simulink model "Battery_Dataset_Generator"  (R2024b)
settings: Solver=FixedStepDiscrete  StartTime=0.0  StopTime=25000  FixedStep=1  RelTol=1e-3
libraries: simulink x1
settings Model: Creator=karth  LastModifiedBy=karth

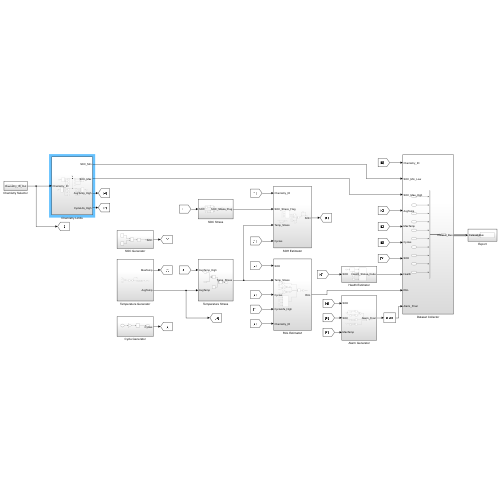
[thumbnail: Simulink's stored preview of the top-level diagram]
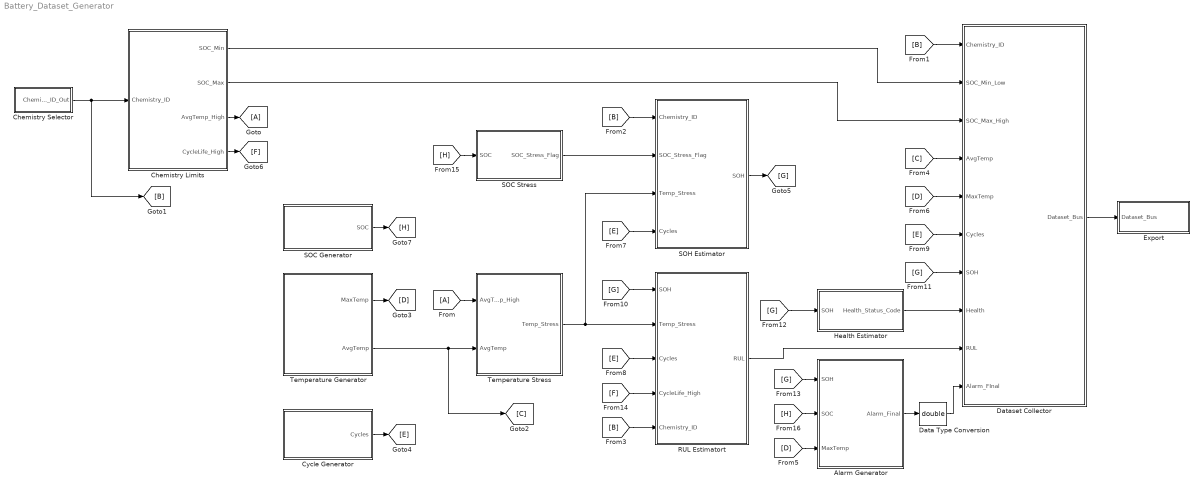
== system Battery_Dataset_Generator ==
  Alarm Generator : Subsystem
  Chemistry Limits : Subsystem
  Chemistry Selector : Subsystem
  Cycle Generator : Subsystem
  Data Type Conversion : DataTypeConversion  OutDataTypeStr=double  SaturateOnIntegerOverflow=off  RndMeth=Floor
  Dataset Collector : Subsystem
  Export : Subsystem
  From : From
  Goto : Goto
  Health Estimator : Subsystem
  RUL Estimatort : Subsystem
  SOC Generator : Subsystem
  SOC Stress : Subsystem
  SOH Estimator : Subsystem
  Temperature Generator : Subsystem
  Temperature Stress : Subsystem
  wires:
  Dataset Collector/1(Dataset_Bus) -> Export/1(Dataset_Bus)
  Chemistry Selector/1(Chemistry_ID_Out) -> Chemistry Limits/1(Chemistry_ID), [B]
  SOC Stress/1(SOC_Stress_Flag) -> SOH Estimator/2(SOC_Stress_Flag)
  Temperature Stress/1(Temp_Stress) -> SOH Estimator/3(Temp_Stress), RUL Estimatort/2(Temp_Stress)
  Chemistry Limits/1(SOC_Min) -> Dataset Collector/2(SOC_Min_Low)
  Chemistry Limits/2(SOC_Max) -> Dataset Collector/3(SOC_Max_High)
  Temperature Generator/2(AvgTemp) -> [C], Temperature Stress/2(AvgTemp)
  RUL Estimatort/1(RUL) -> Dataset Collector/9(RUL)
  Health Estimator/1(Health_Status_Code) -> Dataset Collector/8(Health)
  Chemistry Limits/3(AvgTemp_High) -> Goto/1
  From/1 -> Temperature Stress/1(AvgTemp_High)
  [B] -> SOH Estimator/1(Chemistry_ID)
  [B] -> Dataset Collector/1(Chemistry_ID)
  [C] -> Dataset Collector/4(AvgTemp)
  Temperature Generator/1(MaxTemp) -> [D]
  [D] -> Alarm Generator/3(MaxTemp)
  [D] -> Dataset Collector/5(MaxTemp)
  Cycle Generator/1(Cycles) -> [E]
  [E] -> SOH Estimator/4(Cycles)
  [E] -> RUL Estimatort/3(Cycles)
  [E] -> Dataset Collector/6(Cycles)
  [B] -> RUL Estimatort/5(Chemistry_ID)
  SOH Estimator/1(SOH) -> [G]
  [G] -> Dataset Collector/7(SOH)
  [G] -> Alarm Generator/1(SOH)
  [G] -> Health Estimator/1(SOH)
  [G] -> RUL Estimatort/1(SOH)
  Chemistry Limits/4(CycleLife_High) -> [F]
  [F] -> RUL Estimatort/4(CycleLife_High)
  SOC Generator/1(SOC) -> [H]
  [H] -> SOC Stress/1(SOC)
  [H] -> Alarm Generator/2(SOC)
  Alarm Generator/1(Alarm_Final) -> Data Type Conversion/1
  Data Type Conversion/1 -> Dataset Collector/10(Alarm_FInal)

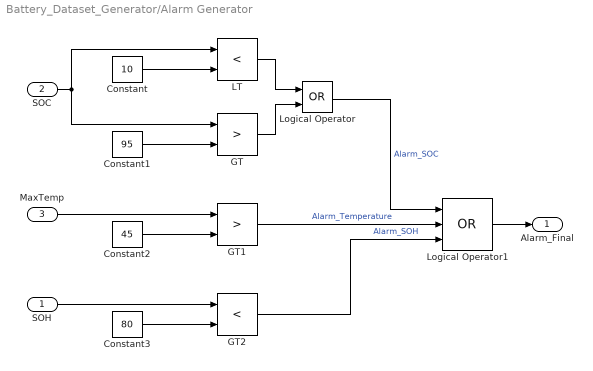
== system Battery_Dataset_Generator/Alarm Generator ==
  SOH : Inport
  SOC : Inport  Port=2
  MaxTemp : Inport  Port=3
  Constant : Constant  Value=10
  Constant1 : Constant  Value=95
  Constant2 : Constant  Value=45
  Constant3 : Constant  Value=80
  GT : RelationalOperator  Operator=>  OutDataTypeStr=boolean  RndMeth=Simplest  InputSameDT=off
  GT1 : RelationalOperator  Operator=>  OutDataTypeStr=boolean  RndMeth=Simplest  InputSameDT=off
  GT2 : RelationalOperator  Operator=<  OutDataTypeStr=boolean  RndMeth=Simplest  InputSameDT=off
  LT : RelationalOperator  Operator=<  OutDataTypeStr=boolean  RndMeth=Simplest  InputSameDT=off
  Logical Operator : Logic  Operator=OR  AllPortsSameDT=off  OutDataTypeStr=boolean
  Logical Operator1 : Logic  Operator=OR  Inputs=3  AllPortsSameDT=off  OutDataTypeStr=boolean
  Alarm_Final : Outport
  wires:
  Constant1/1 -> GT/2
  LT/1 -> Logical Operator/1
  GT/1 -> Logical Operator/2
  SOC/1 -> GT/1, LT/1
  Logical Operator/1 -> Logical Operator1/1  "Alarm_SOC"
  Constant/1 -> LT/2
  GT1/1 -> Logical Operator1/2  "Alarm_Temperature"
  Constant2/1 -> GT1/2
  MaxTemp/1 -> GT1/1
  Constant3/1 -> GT2/2
  GT2/1 -> Logical Operator1/3  "Alarm_SOH"
  SOH/1 -> GT2/1
  Logical Operator1/1 -> Alarm_Final/1

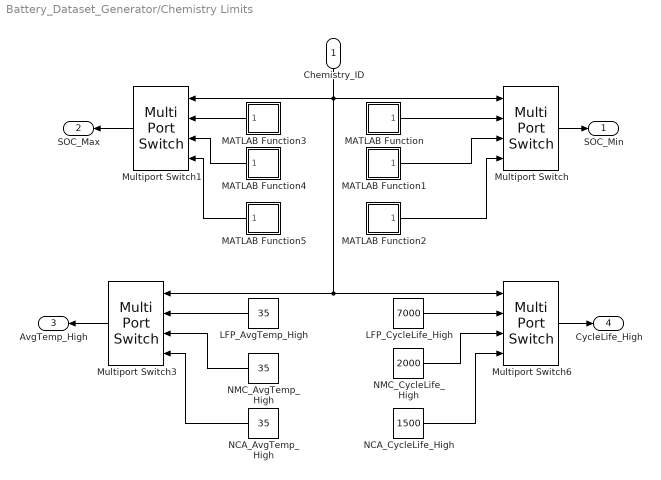
== system Battery_Dataset_Generator/Chemistry Limits ==
  Chemistry_ID : Inport
  LFP_AvgTemp_High : Constant  Value=35
  LFP_CycleLife_High : Constant  Value=7000
  MATLAB Function : MATLAB Function  TreatAsAtomicUnit=on
  MATLAB Function1 : MATLAB Function  TreatAsAtomicUnit=on
  MATLAB Function2 : MATLAB Function  TreatAsAtomicUnit=on
  MATLAB Function3 : MATLAB Function  TreatAsAtomicUnit=on
  MATLAB Function4 : MATLAB Function  TreatAsAtomicUnit=on
  MATLAB Function5 : MATLAB Function  TreatAsAtomicUnit=on
  Multiport Switch{,1,3,6} (4 alike) : MultiPortSwitch  SaturateOnIntegerOverflow=off  InputSameDT=off
  NCA_AvgTemp_High : Constant  Value=35
  NCA_CycleLife_High : Constant  Value=1500
  NMC_AvgTemp_High : Constant  Value=35
  NMC_CycleLife_High : Constant  Value=2000
  SOC_Min : Outport
  SOC_Max : Outport  Port=2
  AvgTemp_High : Outport  Port=3
  CycleLife_High : Outport  Port=4
  wires:
  Multiport Switch/1 -> SOC_Min/1
  Multiport Switch1/1 -> SOC_Max/1
  Multiport Switch3/1 -> AvgTemp_High/1
  MATLAB Function/1(soc_max) -> Multiport Switch/2
  MATLAB Function1/1(soc_max) -> Multiport Switch/3
  MATLAB Function2/1(soc_max) -> Multiport Switch/4
  Chemistry_ID/1 -> Multiport Switch6/1, Multiport Switch3/1, Multiport Switch1/1, Multiport Switch/1
  NCA_AvgTemp_High/1 -> Multiport Switch3/4
  NMC_AvgTemp_High/1 -> Multiport Switch3/3
  LFP_AvgTemp_High/1 -> Multiport Switch3/2
  NMC_CycleLife_High/1 -> Multiport Switch6/3
  Multiport Switch6/1 -> CycleLife_High/1
  LFP_CycleLife_High/1 -> Multiport Switch6/2
  NCA_CycleLife_High/1 -> Multiport Switch6/4
  MATLAB Function3/1(soc_min) -> Multiport Switch1/2
  MATLAB Function4/1(soc_min) -> Multiport Switch1/3
  MATLAB Function5/1(soc_min) -> Multiport Switch1/4

== system Battery_Dataset_Generator/Chemistry Selector ==
  Chemistry_Profile : FromWorkspace  VariableName=chem_profile  SampleTime=1
  Chemistry_ID_Out : Outport
  wires:
  Chemistry_Profile/1 -> Chemistry_ID_Out/1

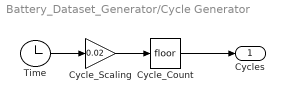
== system Battery_Dataset_Generator/Cycle Generator ==
  Cycle_Count : Rounding
  Cycle_Scaling : Gain  Gain=0.02
  Time : Clock
  Cycles : Outport
  wires:
  Time/1 -> Cycle_Scaling/1
  Cycle_Scaling/1 -> Cycle_Count/1
  Cycle_Count/1 -> Cycles/1

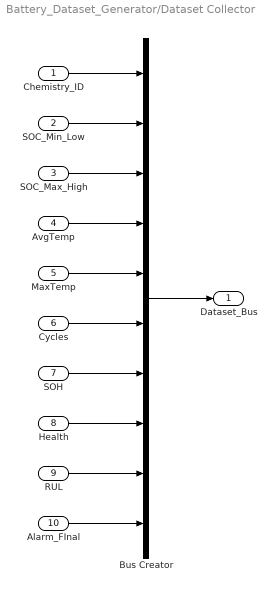
== system Battery_Dataset_Generator/Dataset Collector ==
  Chemistry_ID : Inport
  SOC_Min_Low : Inport  Port=2
  SOC_Max_High : Inport  Port=3
  AvgTemp : Inport  Port=4
  MaxTemp : Inport  Port=5
  Cycles : Inport  Port=6
  SOH : Inport  Port=7
  Health : Inport  Port=8
  RUL : Inport  Port=9
  Alarm_FInal : Inport  Port=10
  Bus Creator : BusCreator  Inputs=10
  Dataset_Bus : Outport
  wires:
  Chemistry_ID/1 -> Bus Creator/1
  SOC_Min_Low/1 -> Bus Creator/2
  SOC_Max_High/1 -> Bus Creator/3
  AvgTemp/1 -> Bus Creator/4
  MaxTemp/1 -> Bus Creator/5
  Cycles/1 -> Bus Creator/6
  SOH/1 -> Bus Creator/7
  Health/1 -> Bus Creator/8
  RUL/1 -> Bus Creator/9
  Alarm_FInal/1 -> Bus Creator/10
  Bus Creator/1 -> Dataset_Bus/1

== system Battery_Dataset_Generator/Export ==
  Dataset_Bus : Inport
  To Workspace : ToWorkspace  VariableName=evbattery  SaveFormat=Structure With Time  SampleTime=1
  wires:
  Dataset_Bus/1 -> To Workspace/1

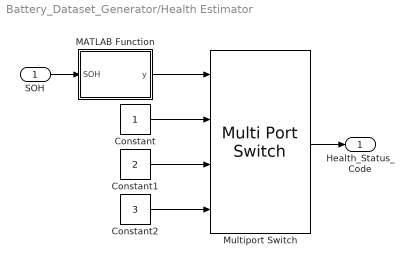
== system Battery_Dataset_Generator/Health Estimator ==
  SOH : Inport
  Constant : Constant
  Constant1 : Constant  Value=2
  Constant2 : Constant  Value=3
  MATLAB Function : MATLAB Function  TreatAsAtomicUnit=on
  Multiport Switch : MultiPortSwitch  SaturateOnIntegerOverflow=off  InputSameDT=off
  Health_Status_Code : Outport
  wires:
  SOH/1 -> MATLAB Function/1(SOH)
  MATLAB Function/1(y) -> Multiport Switch/1
  Constant/1 -> Multiport Switch/2
  Constant1/1 -> Multiport Switch/3
  Constant2/1 -> Multiport Switch/4
  Multiport Switch/1 -> Health_Status_Code/1

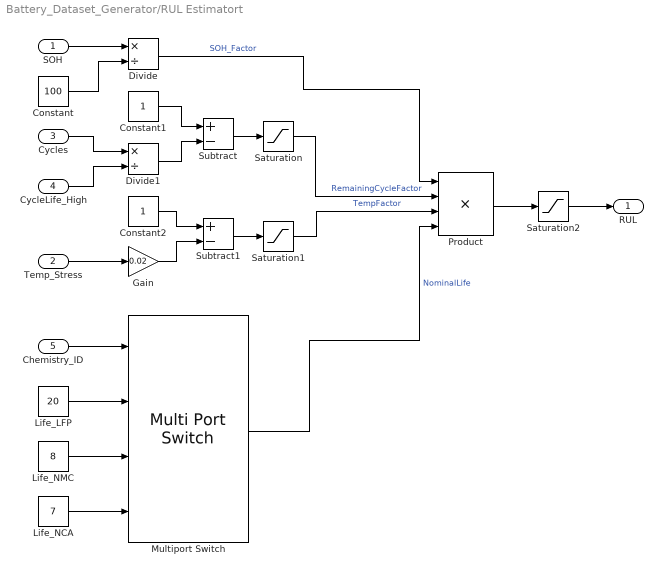
== system Battery_Dataset_Generator/RUL Estimatort ==
  SOH : Inport
  Temp_Stress : Inport  Port=2
  Cycles : Inport  Port=3
  CycleLife_High : Inport  Port=4
  Chemistry_ID : Inport  Port=5
  Constant : Constant  Value=100
  Constant1 : Constant
  Constant2 : Constant
  Divide : Product  Inputs=*/
  Divide1 : Product  Inputs=*/
  Gain : Gain  Gain=0.02
  Life_LFP : Constant  Value=20
  Life_NCA : Constant  Value=7
  Life_NMC : Constant  Value=8
  Multiport Switch : MultiPortSwitch  SaturateOnIntegerOverflow=off  InputSameDT=off
  Product : Product  Inputs=4  OutDataTypeStr=double
  Saturation : Saturate  UpperLimit=1  LowerLimit=0
  Saturation1 : Saturate  UpperLimit=1  LowerLimit=0
  Saturation2 : Saturate  UpperLimit=25  LowerLimit=0
  Subtract : Sum  Inputs=+-
  Subtract1 : Sum  Inputs=+-
  RUL : Outport  SampleTime=1
  wires:
  SOH/1 -> Divide/1
  Constant/1 -> Divide/2
  Divide/1 -> Product/1  "SOH_Factor"
  Cycles/1 -> Divide1/1
  CycleLife_High/1 -> Divide1/2
  Constant1/1 -> Subtract/1
  Divide1/1 -> Subtract/2
  Subtract/1 -> Saturation/1
  Saturation/1 -> Product/2  "RemainingCycleFactor"
  Temp_Stress/1 -> Gain/1
  Constant2/1 -> Subtract1/1
  Gain/1 -> Subtract1/2
  Subtract1/1 -> Saturation1/1
  Life_NMC/1 -> Multiport Switch/3
  Life_NCA/1 -> Multiport Switch/4
  Life_LFP/1 -> Multiport Switch/2
  Chemistry_ID/1 -> Multiport Switch/1
  Multiport Switch/1 -> Product/4  "NominalLife"
  Saturation1/1 -> Product/3  "TempFactor"
  Product/1 -> Saturation2/1
  Saturation2/1 -> RUL/1

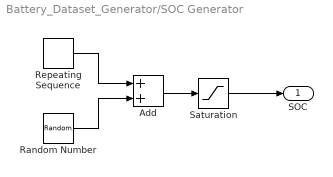
== system Battery_Dataset_Generator/SOC Generator ==
  Add : Sum
  Random Number : RandomNumber  SampleTime=1
  Repeating Sequence : simulink/Sources/Repeating Sequence  rep_seq_t=[0 20 40 60 80 100]  rep_seq_y=[90 70 40 80 30 90]
  Saturation : Saturate  UpperLimit=100  LowerLimit=0
  SOC : Outport
  wires:
  Repeating Sequence/1 -> Add/1
  Random Number/1 -> Add/2
  Add/1 -> Saturation/1
  Saturation/1 -> SOC/1

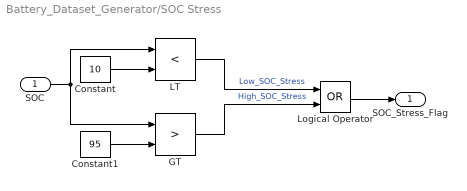
== system Battery_Dataset_Generator/SOC Stress ==
  SOC : Inport
  Constant : Constant  Value=10
  Constant1 : Constant  Value=95
  GT : RelationalOperator  Operator=>  OutDataTypeStr=boolean  RndMeth=Simplest  InputSameDT=off
  LT : RelationalOperator  Operator=<  OutDataTypeStr=boolean  RndMeth=Simplest  InputSameDT=off
  Logical Operator : Logic  Operator=OR  AllPortsSameDT=off  OutDataTypeStr=boolean
  SOC_Stress_Flag : Outport
  wires:
  Constant/1 -> LT/2
  Logical Operator/1 -> SOC_Stress_Flag/1
  Constant1/1 -> GT/2
  GT/1 -> Logical Operator/2  "High_SOC_Stress"
  LT/1 -> Logical Operator/1  "Low_SOC_Stress"
  SOC/1 -> LT/1, GT/1

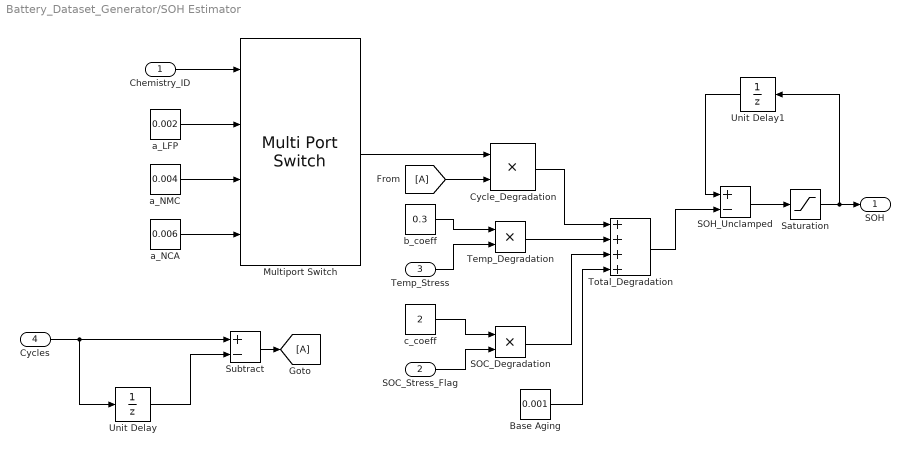
== system Battery_Dataset_Generator/SOH Estimator ==
  Chemistry_ID : Inport
  SOC_Stress_Flag : Inport  Port=2
  Temp_Stress : Inport  Port=3
  Cycles : Inport  Port=4
  Base Aging : Constant  Value=0.001
  Cycle_Degradation : Product
  From : From
  Goto : Goto
  Multiport Switch : MultiPortSwitch  SaturateOnIntegerOverflow=off  InputSameDT=off
  SOC_Degradation : Product
  SOH_Unclamped : Sum  Inputs=+-
  Saturation : Saturate  UpperLimit=100  LowerLimit=0
  Subtract : Sum  Inputs=+-
  Temp_Degradation : Product
  Total_Degradation : Sum  Inputs=++++
  Unit Delay : UnitDelay  SampleTime=-1  HasFrameUpgradeWarning=on
  Unit Delay1 : UnitDelay  InitialCondition=100  HasFrameUpgradeWarning=on
  a_LFP : Constant  Value=0.002
  a_NCA : Constant  Value=0.006
  a_NMC : Constant  Value=0.004
  b_coeff : Constant  Value=0.3
  c_coeff : Constant  Value=2
  SOH : Outport
  wires:
  a_LFP/1 -> Multiport Switch/2
  a_NMC/1 -> Multiport Switch/3
  a_NCA/1 -> Multiport Switch/4
  Chemistry_ID/1 -> Multiport Switch/1
  Multiport Switch/1 -> Cycle_Degradation/1
  b_coeff/1 -> Temp_Degradation/1
  Temp_Stress/1 -> Temp_Degradation/2
  c_coeff/1 -> SOC_Degradation/1
  SOC_Stress_Flag/1 -> SOC_Degradation/2
  Temp_Degradation/1 -> Total_Degradation/2
  Cycle_Degradation/1 -> Total_Degradation/1
  SOC_Degradation/1 -> Total_Degradation/3
  Unit Delay1/1 -> SOH_Unclamped/1
  Total_Degradation/1 -> SOH_Unclamped/2
  SOH_Unclamped/1 -> Saturation/1
  Saturation/1 -> Unit Delay1/1, SOH/1
  Cycles/1 -> Unit Delay/1, Subtract/1
  Unit Delay/1 -> Subtract/2
  Subtract/1 -> Goto/1
  From/1 -> Cycle_Degradation/2
  Base Aging/1 -> Total_Degradation/4

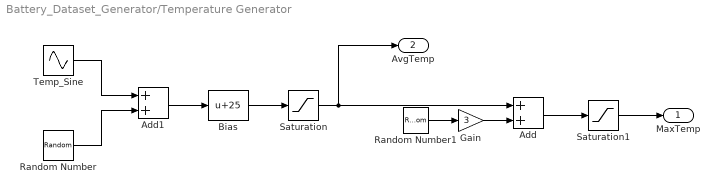
== system Battery_Dataset_Generator/Temperature Generator ==
  Add : Sum
  Add1 : Sum
  Bias : Bias  Bias=25  SaturateOnIntegerOverflow=off
  Gain : Gain  Gain=3
  Random Number : RandomNumber  SampleTime=1
  Random Number1 : RandomNumber  Mean=2  Variance=2  SampleTime=1
  Saturation : Saturate  UpperLimit=60  LowerLimit=0
  Saturation1 : Saturate  UpperLimit=70  LowerLimit=0
  Temp_Sine : Sin  Amplitude=8  Frequency=0.05  SampleTime=1
  MaxTemp : Outport
  AvgTemp : Outport  Port=2
  wires:
  Temp_Sine/1 -> Add1/1
  Random Number/1 -> Add1/2
  Add1/1 -> Bias/1
  Bias/1 -> Saturation/1
  Saturation/1 -> AvgTemp/1, Add/1
  Add/1 -> Saturation1/1
  Random Number1/1 -> Gain/1
  Gain/1 -> Add/2
  Saturation1/1 -> MaxTemp/1

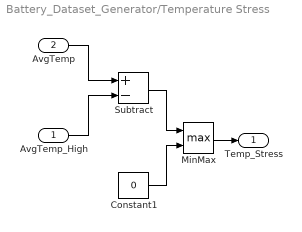
== system Battery_Dataset_Generator/Temperature Stress ==
  AvgTemp_High : Inport
  AvgTemp : Inport  Port=2
  Constant1 : Constant  Value=0
  MinMax : MinMax  Function=max  Inputs=2
  Subtract : Sum  Inputs=+-
  Temp_Stress : Outport
  wires:
  AvgTemp/1 -> Subtract/1
  AvgTemp_High/1 -> Subtract/2
  Subtract/1 -> MinMax/1
  Constant1/1 -> MinMax/2
  MinMax/1 -> Temp_Stress/1

== matlab function Battery_Dataset_Generator/Health Estimator/MATLAB Function ==
  data: SOH input; y output
function y = fcn(SOH)

if SOH < 70
    y = 3;      % EOL
elseif SOH < 80
    y = 2;      % Warning
else
    y = 1;      % Good
end

end

== matlab function Battery_Dataset_Generator/Chemistry Limits/MATLAB Function1 ==
  data: soc_max output
function soc_max = fcn()

soc_max = randi([5,25]);

end

== matlab function Battery_Dataset_Generator/Chemistry Limits/MATLAB Function2 ==
  data: soc_max output
function soc_max = fcn()

soc_max = randi([5,25]);

end

== matlab function Battery_Dataset_Generator/Chemistry Limits/MATLAB Function3 ==
  data: soc_min output
function soc_min = fcn()

soc_min = randi([75,95]);

end

== matlab function Battery_Dataset_Generator/Chemistry Limits/MATLAB Function4 ==
  data: soc_min output
function soc_min = fcn()

soc_min = randi([75,95]);

end

== matlab function Battery_Dataset_Generator/Chemistry Limits/MATLAB Function5 ==
  data: soc_min output
function soc_min = fcn()

soc_min = randi([75,95]);

end

== matlab function Battery_Dataset_Generator/Chemistry Limits/MATLAB Function ==
  data: soc_max output
function soc_max = fcn()

soc_max = randi([5,25]);

end
